simulink model "Custom_SP_inverse"  (R2020b)
settings: Solver=ode45  StartTime=0.0  StopTime=40  RelTol=1e-3
model workspace (MATLAB code in the model file):
  | %% PARAMETERS FOR CUSTOM_SP
  | %%%%%%%%%%%%%%%%%%%%% DENSITY %%%%%%%%%%%%%%%%%%%%%%%
  | al = 2.07; % g/cm^3
  | steel = 7.833; %g/cm^3
  | 
  | %%%%%%%%%%%%%%%%%%%%% BASE COORDINATES %%%%%%%%%%%%%%%%%%%%%%%
  | % Outside coordinates
  | out_base_right = [-335 -170.32; -315 -204.96;
  |     -315 -295.6; -98.49 -420.6; -20 -375.28;
  |     20 -375.28; 315 -204.96; 335 -170.32; 413.49 -125];
  | out_base_left = [413.49 125; 335 170.32;
  |     315 204.96; 20 375.28; -20 375.28;
  |     -98.49 420.6; -315 295.6; -315 204.96; -335 170.32;
  |     -335 -170.32];
  | out_base = [out_base_right; out_base_left];
  | 
  | % Inside coordinates
  | in_base = [-230 -246.52; -230 246.52; -98.49 322.45; 328.49 75.93;
  |     328.49 -75.93; -98.49 -322.45; -230 -246.52];
  | 
  | tot_base = [out_base; in_base];
  | 
  | %%%%%%%%%%%%%%%%%%%%%%% PLATE POSE ON BASE %%%%%%%%%%%%%%%%%%%%%%%%%%%
  | % PLATE POSITION ON BASE
  | plate_1 = [-272.22 -252.09 0];
  | plate_2 = [-82.21 -361.79 0];
  | plate_3 = [354.42 -109.71 0];
  | plate_4 = [354.42 109.71 0];
  | plate_5 = [-82.21 361.79 0];
  | plate_6 = [-272.22  252.09 0];
  | 
  | % ANGLE FOR JOINT ON BASE
  | plate_angle_1 = 0 + pi/2;
  | plate_angle_2 = 2*pi/3 + pi/2;
  | plate_angle_3 = 2*pi/3 + pi/2;
  | plate_angle_4 = 4*pi/3 + pi/2;
  | plate_angle_5 = 4*pi/3 + pi/2;
  | plate_angle_6 = 0 + pi/2;
  | 
  | %%%%%%%%%%%%%%%%%%%%%%%% FLANGE COORDINATES %%%%%%%%%%%%%%%%%%%%%%%%%%%%
  | flange_body = [ -20 22.5; -20 -22.5; 13.6488 -9.3106];
  | 
  | C = linspace(-68.6, 68.6, 21)';
  | C = deg2rad(C);
  | flange_round = [10+10*cos(C) 10*sin(C)];
  | 
  | C = linspace(3*pi/2, -pi/2, 100)';
  | flange_hole = [10+6*cos(C) 6*sin(C)];
  | 
  | flange = [flange_round; flange_body; flange_hole];
  | 
  | %plot(flange(:,1),flange(:,2), 'Color', [0.6 0.6 0.6], 'Marker', '.',...
  | %'MarkerSize', 9, 'MarkerEdgeColor', [1 0 0]);
  | 
  | %%%%%%%%%%%%%%%%%%%%%%%%%%%%% LID %%%%%%%%%%%%%%%%%%%%%%%%%%%%%%
  | % LID COORDINATES
  | C = linspace(-150 , -70, 9)';
  | C = deg2rad(C);
  | lid_round1 = [-171.37+10*cos(C) -103.18+10*sin(C)];
  | 
  | C = linspace(110, 60, 9)';
  | C = deg2rad(C);
  | lid_round2 = [-118.05+10*cos(C) -105.05+10*sin(C)];
  | 
  | C = linspace(60, 10, 9)';
  | C = deg2rad(C);
  | lid_round3 = [-117.46+10*cos(C) -105.39+10*sin(C)];
  | 
  | C = linspace(110, 60, 9)';
  | C = deg2rad(C);
  | lid_round4 = [-32.54+10*cos(C) -154.42+10*sin(C)];
  | 
  | C = linspace(60, 10, 9)';
  | C = deg2rad(C);
  | lid_round5 = [-31.95+10*cos(C) -154.76+10*sin(C)];
  | 
  | C = linspace(-90-80, -90, 9)';
  | C = deg2rad(C);
  | lid_round6 = [-3.67+10*cos(C) -200+10*sin(C)];
  | 
  | C = linspace(-30, 50, 9)';
  | C = deg2rad(C);
  | lid_round7 = [175.04+10*cos(C) -96.82+10*sin(C)];
  | 
  | C = linspace(-140, -90, 9)';
  | C = deg2rad(C);
  | lid_round8 = [150+10*sin(C) -49.71+10*cos(C)];
  | 
  | C = linspace(-90, -40, 9)';
  | C = deg2rad(C);
  | lid_round9 = [150+10*sin(C) -49.03+10*cos(C)];
  | 
  | C = linspace(-140, -90, 9)';
  | C = deg2rad(C);
  | lid_round10 = [150+10*sin(C) 49.03+10*cos(C)];
  | 
  | C = linspace(-90, -40, 9)';
  | C = deg2rad(C);
  | lid_round11 = [150+10*sin(C) 49.71+10*cos(C)];
  | 
  | C = linspace(-50, 30, 9)';
  | C = deg2rad(C);
  | lid_round12 = [175.04+10*cos(C) 96.82+10*sin(C)];
  | 
  | C = linspace(90, 90+80, 9)';
  | C = deg2rad(C);
  | lid_round13 = [-3.67+10*cos(C) 200+10*sin(C)];
  | 
  | C = linspace(-10, -60, 9)';
  | C = deg2rad(C);
  | lid_round14 = [-31.95+10*cos(C) 154.76+10*sin(C)];
  | 
  | C = linspace(-60, -110, 9)';
  | C = deg2rad(C);
  | lid_round15 = [-32.54+10*cos(C) 154.42+10*sin(C)];
  | 
  | C = linspace(-10, -60, 9)';
  | C = deg2rad(C);
  | lid_round16 = [-117.46+10*cos(C) 105.39+10*sin(C)];
  | 
  | C = linspace(-60, -110, 9)';
  | C = deg2rad(C);
  | lid_round17 = [-118.05+10*cos(C) 105.05+10*sin(C)];
  | 
  | C = linspace(70 , 150, 9)';
  | C = deg2rad(C);
  | lid_round18 = [-171.37+10*cos(C) 103.18+10*sin(C)];
  | 
  | lid = [-200 -73.59; lid_round1; lid_round2;
  |     lid_round3;
  |     -100.49 -144.05; -74.51 -159.05; lid_round4;
  |     lid_round5; lid_round6; 36.27 -210; 163.73 -136.41;
  |     lid_round7; lid_round8; lid_round9; 175 -15; 175 15;
  |     lid_round10; lid_round11; lid_round12; 163.73 136.41;
  |     36.27 210; lid_round13; lid_round14; lid_round15;
  |     -74.51 159.05; -100.49 144.05; lid_round16;
  |     lid_round17; lid_round18; -200 73.59];
  | 
  | lid = [-200 -73.59; lid_round1; lid_round2; lid_round3;
  |     -100.49 -144.05; -74.51 -159.05;
  |     lid_round4; lid_round5; lid_round6;
  |     36.27 -210; 163.73 -136.41;
  |     lid_round7; lid_round8; lid_round9;
  |     175 -15; 175 15;
  |     lid_round10; lid_round11; lid_round12;
  |     163.73 136.41; 36.27 210;
  |     lid_round13; lid_round14; lid_round15;
  |     -74.51 159.05; -100.49 144.05;
  |     lid_round16; lid_round17; lid_round18; -200 73.59];
  | 
  | % LID CONNECTOR
  | C = linspace(-150 , -50, 15)';
  | C = deg2rad(C);
  | lid_connector_round1 = [2.15+10*cos(C) -79.37+10*sin(C)];
  | 
  | C = linspace(-50 , 0, 15)';
  | C = deg2rad(C);
  | lid_connector_round2 = [37.5+10*cos(C) -49.71+10*sin(C)];
  | 
  | C = linspace(0 , 50, 15)';
  | C = deg2rad(C);
  | lid_connector_round3 = [37.5+10*cos(C) -49.03+10*sin(C)];
  | 
  | C = linspace(-50, 0, 15)';
  | C = deg2rad(C);
  | lid_connector_round4 = [37.5+10*cos(C) 49.03+10*sin(C)];
  | 
  | C = linspace(0, 50, 15)';
  | C = deg2rad(C);
  | lid_connector_round5 = [37.5+10*cos(C) 49.71+10*sin(C)];
  | 
  | C = linspace(50 , 150, 15)';
  | C = deg2rad(C);
  | lid_connector_round6 = [2.15+10*cos(C) 79.37+10*sin(C)];
  | 
  | lid_connector = [-12.5 -74; lid_connector_round1;
  |     lid_connector_round2; lid_connector_round3; 12.5 -15;
  |     12.5 15; lid_connector_round4; lid_connector_round5;
  |     lid_connector_round6; -12.5 74];
  | 
  | %%%%%%%%%%%%%%%%%%%%%%%%% BALL JOINT %%%%%%%%%%%%%%%%%%%%%%%%%%%
  | % BALL JOINTS
  | C = linspace(138.59, 41.41, 50)';
  | C = deg2rad(C);
  | ball_round = [10*sin(C) 10*cos(C)];
  | 
  | ball_joint = [6 -7.5; ball_round; 6 7.5];
  | 
  | % BALL CONNECTOR
  | C = linspace(-109.47, -70.53, 49)';
  | C = deg2rad(C);
  | ball_round_out = [-16*sin(C) 16*cos(C)];
  | 
  | C = linspace(-57.75, -122.25, 49)';
  | C = deg2rad(C);
  | ball_round_in = [-10*sin(C) 10*cos(C)];
  | 
  | ball_connector = [ball_round_out; ball_round_in];
  | 
  | %%%%%%%%%%%%%%%%%%%%%%%%%% MOTOR %%%%%%%%%%%%%%%%%%%%%%%%%%%
  | % KNOB UNDER MOTOR
  | C = linspace(-90+25.84, -90+64.16, 50)';
  | C = deg2rad(C);
  | knob_under_round1 = [7.5*sin(C) -7.5*cos(C)];
  | 
  | C = linspace( -64.16, -25.84, 50)';
  | C = deg2rad(C);
  | knob_under_round2 = [7.5*cos(C) 7.5*sin(C)];
  | 
  | C = linspace( 25.84, 64.16, 50)';
  | C = deg2rad(C);
  | knob_under_round3 = [7.5*cos(C) 7.5*sin(C)];
  | 
  | C = linspace( 64.16, 25.84, 50)';
  | C = deg2rad(C);
  | knob_under_round4 = [-7.5*cos(C) 7.5*sin(C)];
  | 
  | knob_under = [knob_under_round1; knob_under_round2;
  |     knob_under_round3; knob_under_round4];
  | 
  | % MOTOR UNDER
  | C = linspace(-90, -49, 10)';
  | C = deg2rad(C);
  | knob_under_round1 = [-(19+17)+5.5*sin(C) -11.13-5.5*cos(C)];
  | 
  | C = linspace(-49, 0, 10)';
  | C = deg2rad(C);
  | knob_under_round2 = [-(17+14.77)+5.5*sin(C) -16-5.5*cos(C)];
  | 
  | C = linspace(0, 180, 49)';
  | C = deg2rad(C);
  | knob_under_round3 = [20+21.5*sin(C) -21.5*cos(C)];
  | 
  | C = linspace(180, 180+49, 10)';
  | C = deg2rad(C);
  | knob_under_round4 = [-(17+14.77)+5.5*sin(C) 16-5.5*cos(C)];
  | 
  | C = linspace(270-49, 270, 10)';
  | C = deg2rad(C);
  | knob_under_round5 = [-(19+17)+5.5*sin(C) 11.13-5.5*cos(C)];
  | 
  | motor_under = [knob_under_round1; knob_under_round2;
  |     knob_under_round3; knob_under_round4; knob_under_round5];
  | 
  | % MOTOR LINEAR
  | C = linspace(-180, -101.99, 10)';
  | C = deg2rad(C);
  | motor_top_round1 = [-15.28+3*cos(C) -8.62+3*sin(C)];
  | 
  | C = linspace(-101.99, 101.99, 49)';
  | C = deg2rad(C);
  | motor_top_round2 = [3.12+15.25*cos(C) 15.25*sin(C)];
  | 
  | C = linspace(101.99, 180, 10)';
  | C = deg2rad(C);
  | motor_top_round3 = [-15.28+3*cos(C) 8.62+3*sin(C)];
  | 
  | C = linspace(180, -180, 50)';
  | C = deg2rad(C);
  | motor_top_hole = [3.12+10.1*cos(C) 10.1*sin(C)];
  | 
  | motor_linear = [motor_top_round1; motor_top_round2; motor_top_round3;
  |     -15.28-3 -8.62; motor_top_hole];
  | 
  | %%%%%%%%%%%%%%%%%%%%% MALE %%%%%%%%%%%%%%%%%%%%%%%%%%%
  | male = [15.1 -16; 15.1 16; 10.1 16;
  |     10.1 -11; 6 -11; 6 -16];
  | 
  | %%%%%%%%%%%%%%%%%%%%% FEMALE %%%%%%%%%%%%%%%%%%%%%%%%%
  | female = [15 -19; 15 19; 9.5 19; 9.5 1;
  |     5.055 1; 5.055 -19];
  | 
  | %%%%%%%%%%%%%%%%%%%%% STRAIN GAUGE %%%%%%%%%%%%%%%%%%%%%%
  | strain_gauge = [-38.1 -25.4; -22.4 -25.4; -22.4 11.6;
  |     -13.9 11.6; -13.9 -25.4; 38.1 -25.4; 38.1 25.4;
  |     22.4 25.4; 22.4 -11.6; 13.9 -11.6;
  |     13.9 25.4; -38.1 25.4];
  | 
  | %%%%%%%%%%%%%%%%%%%%% M12 STUFF %%%%%%%%%%%%%%%%%%%%%%%%%%%
  | % M12 BOLT
  | m12_bolt = [0 -18.5; 6 -18.5; 6 11.5; 10.1 11.5; 10.1 18.5; 0 18.5];
  | 
  | % M12 NUT
  | C = linspace(3*pi, pi, 50)';
  | m12_hole = [6*cos(C) 6*sin(C)];
  | m12_nut = [-21.2/2 0; -5.48 -9.5; 5.48 -9.5; 21.2/2 0; 5.48 9.5; -5.48 9.5; -21.2/2 0; m12_hole];
  | 
  | % M12 WASHER
  | m12_washer = [6 -1; 23.5/2 -1; 23.5/2 1; 6 1];
  | 
  | %%%%%%%%%%%%%%%%%%%%%% PLATFORM COORDINATES %%%%%%%%%%%%%%%%%%%%%%%%%%%
  | % Outside coordinates
  | out_platform = [36.27 -210; 163.73 -136.41;
  |     200 -73.59; 200 73.59; 163.73 136.41;
  |     36.27 210; -36.27 210; -163.73 136.41;
  |     -200 73.59; -200 -73.54; -163.73 -136.41; -36.27 -210;
  |     36.27 -210];
  | C = linspace(3*pi/2, -pi/2, 100)';
  | platform_hole = [140*cos(C) 140*sin(C)];
  | platform = [out_platform; platform_hole];
  | 
  | %%%%%%%%%%%%%%%%%%%% STUMP %%%%%%%%%%%%%%%%%%%%%%%
  | C = linspace(-pi/2, -deg2rad(12.47), 100)';
  | stump_round = [70*cos(C) -100+70*sin(C)];
  | stump = [stump_round; 100 170; 0 170];
  | 
  | %% POSITION OF BASE JOINT AND PLATFORM JOINT FOR INVERSE KINEMATICS
  | % BASE JOINT POSITION
  | 
  | zb = 5 + 5 + 30;
  | B = [plate_1(1,1:2) zb; plate_2(1,1:2) zb; plate_3(1,1:2) zb; plate_4(1,1:2) zb; plate_5(1,1:2) zb; plate_6(1,1:2) zb]';
  | 
  | 
  | % JOINT POSITION ON PLATFORM
  | Rot = [cos(deg2rad(120)) -sin(deg2rad(120)); sin(deg2rad(120)) cos(deg2rad(120))];
  | platform_joint_1 = [-200.54-18.5 -48.83]';
  | platform_joint_6 = [-200.54-18.5 48.83]';
  | platform_joint_2 = Rot*platform_joint_6;
  | platform_joint_3 = Rot*platform_joint_1;
  | platform_joint_4 = Rot*platform_joint_2;
  | platform_joint_5 = Rot*platform_joint_3;
  | 
  | % LEG LENGHT AT HOME POSITION
  | %ball_joint_bottom_length = 13.75; %mm
  | %nut_washer = 10 + 2 + 7.25; %mm
  | %female_length = 38 + 2; %mm
  | %motor_length = 58.5 + 163.5; %mm
  | %extender_length = 20 + 50; %mm
  | %male_bolt_nut = 5 + 7 + 25; %mm
  | %strain_gauge_length = 38.1*2; %mm
  | %nut = 10 + 7.25; %mm
  | %ball_joint_top_length = 13.75; %mm
  | 
  | %leg_initial_length = ball_joint_bottom_length + nut_washer + female_length + motor_length + extender_length + male_bolt_nut + strain_gauge_length + nut + ball_joint_top_length;
  | 
  | %height_home = sqrt(leg_initial_length^2 - (plate_1(1)-platform_joint_1(1))^2 - (plate_1(2)-platform_joint_1(2))^2)+zb;
  | height_home = 503.318 + 2.5;
  | leg_initial_length = sqrt((plate_1(1)-platform_joint_1(1))^2 + (plate_1(2)-platform_joint_1(2))^2 + (height_home-zb)^2);
  | P = [platform_joint_1' height_home; platform_joint_2' height_home; platform_joint_3' height_home; platform_joint_4' height_home; platform_joint_5' height_home; platform_joint_6' height_home]';
libraries: nesl_utility x19, Custom_SP_lib x8, sm_lib x2
(part 2 of 2)

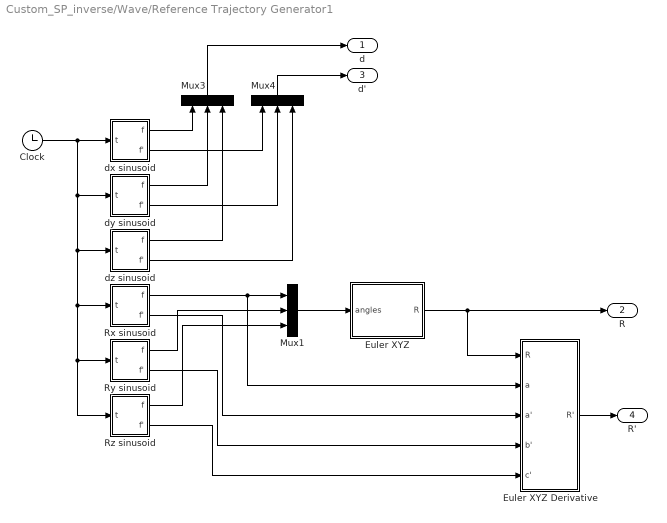
== system Custom_SP_inverse/Wave/Reference Trajectory Generator1 ==
  Clock : Clock
  Euler XYZ : Subsystem  mask(Euler XYZ){}
      mask help: Converts a set of Euler angles to the corresponding rotation matrix from rotated frame to fixed frame coordinates.
      mask Help:
      | An <em>Euler XYZ</em>  block converts a set of Euler angles to the corresponding
      |   rotation matrix from rotated frame to fixed frame coordinates.
      | 
      | Arbitrary 3-D rotations can be parameterized by a vector of three Euler angles:
      |   a, b, and c.  The resulting rotation is given by
      | 
      |     <b>R</b> = <b>R_x</b>(a) <b>R_y</b>(b) <b>R_z</b>(c).
      | 
      | where <b>R_x</b>, <b>R_y</b>, and <b>R_z</b> are rotations about the x, y, and z
      | axes, respectively.
      | 
      | The complete rotation <b>R</b> maps directions from a rotated frame F to a
      | fixed frame G.  Beginning with F and G in an aligned configuration, the full
      | rotation can be realized as a sequence of three rotations: first rotate F
      | about its x-axis, then rotate F about its y-axis, and finally rotate F about its
      | z-axis.  Alternatively, the rotation can be realized in a fixed-frame manner:
      | first rotate F about G's z-axis, then rotate F about G's y-axis, and finally
      | rotate F about G's z-axis.  Both interpretations are correct.
      | 
      | 
      | <h3>Ports</h3>
      | 
      | <ul>
      | 
      | <li> <b>angles</b> The Euler angles a, b, and c (in that order) as a 3-vector
      |   with units of radians.
      | 
      | <li> <b>R</b> The resulting rotation matrix.  This matrix is always a 3 x 3
      | orthogonal matrix with a +1 determinant.
      | 
      | </ul>
  Euler XYZ Derivative : Subsystem  mask(Euler XYZ Derivative){}
      mask help: Computes the first time derivative of a rotation matrix specified by a set of Euler angles.
      mask Help:
      | An <em>Euler XYZ Derivative</em>  block computes the first time derivative of a
      |  rotation matrix specified by a set of Euler angles.
      | 
      | Arbitrary 3-D rotations can be parameterized by a vector of three Euler angles:
      |   a, b, and c.  The resulting rotation is given by
      | 
      |     <b>R</b> = <b>R_x</b>(a) <b>R_y</b>(b) <b>R_z</b>(c).
      | 
      | where <b>R_x</b>, <b>R_y</b>, and <b>R_z</b> are rotations about the x, y, and z
      | axes, respectively.
      | 
      | If a, b, and c are, in turn, functions of time, with instantaneous derivatives
      | a', b', and c', then <b>R'</b>, the time derivative of <b>R</b> is given by
      | 
      |     <b>R'</b> = a' <b>i~ R_x</b>(a) <b>R_y</b>(b) <b>R_z</b>(c) + b' <b>R_x</b>(a) <b>j~ R_y</b>(b) <b>R_z</b>(c) + c' <b>R_x</b>(a) <b>R_y</b>(b) <b>k~ R_z</b>(c),
      | 
      | where <b>~</b> is the canonical operator converting a 3-vector <b>v</b> into a
      | corresponding 3 x 3 skew-symmetric matrix <b>v~</b> such that
      | 
      |     <b>v~ u</b> = <b>v</b> x <b>u</b> for all <b>u</b>.
      | 
      | With some vector algebra, the above expression of <b>R'</b> can be simplified to
      | 
      |     <b>R'</b> = [a' <b>i</b> + b' <b>R_x</b>(a) <b>j</b> ]<b>~</b> <b>R</b> + c' <b>[+R_2, -R_1, 0]</b>
      | 
      | where <b>R_i</b> is the ith column of <b>R</b>.
      | 
      | The block computes the value of <b>R'</b> according to the last equation above.
      | In addition to <b>R</b>, the computation requires the scalar Euler
      | angle <em>a</em>, and the time derivatives of all three Euler angles.
      | 
      | 
      | <h3>Ports</h3>
      | 
      | <ul>
      | 
      | <li> <b>R</b> The rotation matrix defined by the Euler angles <em>a, b,</em>
      | and <em>c</em> (see above).
      | 
      | <li> <b>a</b> The Euler angle corresponding to rotation about the x-axis.
      | 
      | <li> <b>a'</b> The time derivative of the Euler angle corresponding to rotation
      | about the x-axis.
      | 
      | <li> <b>b'</b> The time derivative of the Euler angle corresponding to rotation
      | about the y-axis.
      | 
      | <li> <b>c'</b> The time derivative of the Euler angle corresponding to rotation
      | about the z-axis.
      | 
      | </ul>
  Mux1 : Mux  Inputs=3
  Mux3 : Mux  Inputs=3
  Mux4 : Mux  Inputs=3
  Rx sinusoid : Subsystem  mask(Sinusoidal Trajectory){A=Aa * pi/180, w=wa, p=pa, k=ka * pi/180}
      mask prompts: A "Amplitude"; w "Frequency (deg / s)"; p "Phase (deg)"; k "Offset"
      mask help: Produces a time-varying sinusoid parameterized by amplitude, frequency, phase, and offset. Also produces the first time derivative of this function.
      mask Help:
      | A <em>Sinusoidal Trajectory</em> produces a time-varying sinusoid
      |  parameterized by amplitude, frequency, phase, and offset.  It also produces the
      |  first time derivative of this function.
      | 
      | <h3>Sinsoidal Functions</h3>
      | 
      | An arbitrary sinusoidal function of time and its first time derivative are given by
      | 
      |     f(t) = A sin (w t + p) + k
      |     f'(t) = w A cos (w t + p),
      | 
      | where <em>t</em> is time, and <em>A, w, p,</em> and <em>k</em> are scalar
      | constants.  Given time as an input signal, this block provides the f(t) and
      | f'(t) signals based on the parameters described above.
      | 
      | 
      | <h3>Parameters</h3>
      | 
      | The four parameters specify the scalar parameters described above:
      | 
      | <ul>
      | 
      | <li> <b>A</b> The <em>amplitude</em> of the sinusoid.
      | 
      | <li> <b>w</b> The <em>angular frequency</em> of the sinusoid.
      | 
      | <li> <b>p</b> The <em>phase</em> of the sinusoid.
      | 
      | <li> <b>k</b> The <em>offset</em> of the sinusoid.
      | 
      | </ul>
      | 
      | </ul>
      | 
      | <h3>Ports</h3>
      | 
      | <ul>
      | 
      | <li><b>t</b> The time function, provided as an input signal.
      | 
      | <li><b>f</b> The sinusoid f(t), as described above, as an output signal.
      | 
      | <li><b>f'</b> The sinusoid's first time derivative f'(t), as described above, as an output signal.
      | 
      | </ul>
  Ry sinusoid : Subsystem  mask(Sinusoidal Trajectory){A=Ab * pi/180, w=wb, p=pb, k=kb * pi/180}
      mask prompts: A "Amplitude"; w "Frequency (deg / s)"; p "Phase (deg)"; k "Offset"
      mask help: Produces a time-varying sinusoid parameterized by amplitude, frequency, phase, and offset. Also produces the first time derivative of this function.
      mask Help:
      | A <em>Sinusoidal Trajectory</em> produces a time-varying sinusoid
      |  parameterized by amplitude, frequency, phase, and offset.  It also produces the
      |  first time derivative of this function.
      | 
      | <h3>Sinsoidal Functions</h3>
      | 
      | An arbitrary sinusoidal function of time and its first time derivative are given by
      | 
      |     f(t) = A sin (w t + p) + k
      |     f'(t) = w A cos (w t + p),
      | 
      | where <em>t</em> is time, and <em>A, w, p,</em> and <em>k</em> are scalar
      | constants.  Given time as an input signal, this block provides the f(t) and
      | f'(t) signals based on the parameters described above.
      | 
      | 
      | <h3>Parameters</h3>
      | 
      | The four parameters specify the scalar parameters described above:
      | 
      | <ul>
      | 
      | <li> <b>A</b> The <em>amplitude</em> of the sinusoid.
      | 
      | <li> <b>w</b> The <em>angular frequency</em> of the sinusoid.
      | 
      | <li> <b>p</b> The <em>phase</em> of the sinusoid.
      | 
      | <li> <b>k</b> The <em>offset</em> of the sinusoid.
      | 
      | </ul>
      | 
      | </ul>
      | 
      | <h3>Ports</h3>
      | 
      | <ul>
      | 
      | <li><b>t</b> The time function, provided as an input signal.
      | 
      | <li><b>f</b> The sinusoid f(t), as described above, as an output signal.
      | 
      | <li><b>f'</b> The sinusoid's first time derivative f'(t), as described above, as an output signal.
      | 
      | </ul>
  Rz sinusoid : Subsystem  mask(Sinusoidal Trajectory){A=Ac * pi/180, w=wc, p=pc, k=kc * pi/180}
      mask prompts: A "Amplitude"; w "Frequency (deg / s)"; p "Phase (deg)"; k "Offset"
      mask help: Produces a time-varying sinusoid parameterized by amplitude, frequency, phase, and offset. Also produces the first time derivative of this function.
      mask Help:
      | A <em>Sinusoidal Trajectory</em> produces a time-varying sinusoid
      |  parameterized by amplitude, frequency, phase, and offset.  It also produces the
      |  first time derivative of this function.
      | 
      | <h3>Sinsoidal Functions</h3>
      | 
      | An arbitrary sinusoidal function of time and its first time derivative are given by
      | 
      |     f(t) = A sin (w t + p) + k
      |     f'(t) = w A cos (w t + p),
      | 
      | where <em>t</em> is time, and <em>A, w, p,</em> and <em>k</em> are scalar
      | constants.  Given time as an input signal, this block provides the f(t) and
      | f'(t) signals based on the parameters described above.
      | 
      | 
      | <h3>Parameters</h3>
      | 
      | The four parameters specify the scalar parameters described above:
      | 
      | <ul>
      | 
      | <li> <b>A</b> The <em>amplitude</em> of the sinusoid.
      | 
      | <li> <b>w</b> The <em>angular frequency</em> of the sinusoid.
      | 
      | <li> <b>p</b> The <em>phase</em> of the sinusoid.
      | 
      | <li> <b>k</b> The <em>offset</em> of the sinusoid.
      | 
      | </ul>
      | 
      | </ul>
      | 
      | <h3>Ports</h3>
      | 
      | <ul>
      | 
      | <li><b>t</b> The time function, provided as an input signal.
      | 
      | <li><b>f</b> The sinusoid f(t), as described above, as an output signal.
      | 
      | <li><b>f'</b> The sinusoid's first time derivative f'(t), as described above, as an output signal.
      | 
      | </ul>
  dx sinusoid : Subsystem  mask(Sinusoidal Trajectory){A=Ax, w=wx, p=px, k=kx}
      mask prompts: A "Amplitude"; w "Frequency (deg / s)"; p "Phase (deg)"; k "Offset"
      mask help: Produces a time-varying sinusoid parameterized by amplitude, frequency, phase, and offset. Also produces the first time derivative of this function.
      mask Help:
      | A <em>Sinusoidal Trajectory</em> produces a time-varying sinusoid
      |  parameterized by amplitude, frequency, phase, and offset.  It also produces the
      |  first time derivative of this function.
      | 
      | <h3>Sinsoidal Functions</h3>
      | 
      | An arbitrary sinusoidal function of time and its first time derivative are given by
      | 
      |     f(t) = A sin (w t + p) + k
      |     f'(t) = w A cos (w t + p),
      | 
      | where <em>t</em> is time, and <em>A, w, p,</em> and <em>k</em> are scalar
      | constants.  Given time as an input signal, this block provides the f(t) and
      | f'(t) signals based on the parameters described above.
      | 
      | 
      | <h3>Parameters</h3>
      | 
      | The four parameters specify the scalar parameters described above:
      | 
      | <ul>
      | 
      | <li> <b>A</b> The <em>amplitude</em> of the sinusoid.
      | 
      | <li> <b>w</b> The <em>angular frequency</em> of the sinusoid.
      | 
      | <li> <b>p</b> The <em>phase</em> of the sinusoid.
      | 
      | <li> <b>k</b> The <em>offset</em> of the sinusoid.
      | 
      | </ul>
      | 
      | </ul>
      | 
      | <h3>Ports</h3>
      | 
      | <ul>
      | 
      | <li><b>t</b> The time function, provided as an input signal.
      | 
      | <li><b>f</b> The sinusoid f(t), as described above, as an output signal.
      | 
      | <li><b>f'</b> The sinusoid's first time derivative f'(t), as described above, as an output signal.
      | 
      | </ul>
  dy sinusoid : Subsystem  mask(Sinusoidal Trajectory){A=Ay, w=wy, p=py, k=ky}
      mask prompts: A "Amplitude"; w "Frequency (deg / s)"; p "Phase (deg)"; k "Offset"
      mask help: Produces a time-varying sinusoid parameterized by amplitude, frequency, phase, and offset. Also produces the first time derivative of this function.
      mask Help:
      | A <em>Sinusoidal Trajectory</em> produces a time-varying sinusoid
      |  parameterized by amplitude, frequency, phase, and offset.  It also produces the
      |  first time derivative of this function.
      | 
      | <h3>Sinsoidal Functions</h3>
      | 
      | An arbitrary sinusoidal function of time and its first time derivative are given by
      | 
      |     f(t) = A sin (w t + p) + k
      |     f'(t) = w A cos (w t + p),
      | 
      | where <em>t</em> is time, and <em>A, w, p,</em> and <em>k</em> are scalar
      | constants.  Given time as an input signal, this block provides the f(t) and
      | f'(t) signals based on the parameters described above.
      | 
      | 
      | <h3>Parameters</h3>
      | 
      | The four parameters specify the scalar parameters described above:
      | 
      | <ul>
      | 
      | <li> <b>A</b> The <em>amplitude</em> of the sinusoid.
      | 
      | <li> <b>w</b> The <em>angular frequency</em> of the sinusoid.
      | 
      | <li> <b>p</b> The <em>phase</em> of the sinusoid.
      | 
      | <li> <b>k</b> The <em>offset</em> of the sinusoid.
      | 
      | </ul>
      | 
      | </ul>
      | 
      | <h3>Ports</h3>
      | 
      | <ul>
      | 
      | <li><b>t</b> The time function, provided as an input signal.
      | 
      | <li><b>f</b> The sinusoid f(t), as described above, as an output signal.
      | 
      | <li><b>f'</b> The sinusoid's first time derivative f'(t), as described above, as an output signal.
      | 
      | </ul>
  dz sinusoid : Subsystem  mask(Sinusoidal Trajectory){A=Az, w=wz, p=pz, k=kz}
      mask prompts: A "Amplitude"; w "Frequency (deg / s)"; p "Phase (deg)"; k "Offset"
      mask help: Produces a time-varying sinusoid parameterized by amplitude, frequency, phase, and offset. Also produces the first time derivative of this function.
      mask Help:
      | A <em>Sinusoidal Trajectory</em> produces a time-varying sinusoid
      |  parameterized by amplitude, frequency, phase, and offset.  It also produces the
      |  first time derivative of this function.
      | 
      | <h3>Sinsoidal Functions</h3>
      | 
      | An arbitrary sinusoidal function of time and its first time derivative are given by
      | 
      |     f(t) = A sin (w t + p) + k
      |     f'(t) = w A cos (w t + p),
      | 
      | where <em>t</em> is time, and <em>A, w, p,</em> and <em>k</em> are scalar
      | constants.  Given time as an input signal, this block provides the f(t) and
      | f'(t) signals based on the parameters described above.
      | 
      | 
      | <h3>Parameters</h3>
      | 
      | The four parameters specify the scalar parameters described above:
      | 
      | <ul>
      | 
      | <li> <b>A</b> The <em>amplitude</em> of the sinusoid.
      | 
      | <li> <b>w</b> The <em>angular frequency</em> of the sinusoid.
      | 
      | <li> <b>p</b> The <em>phase</em> of the sinusoid.
      | 
      | <li> <b>k</b> The <em>offset</em> of the sinusoid.
      | 
      | </ul>
      | 
      | </ul>
      | 
      | <h3>Ports</h3>
      | 
      | <ul>
      | 
      | <li><b>t</b> The time function, provided as an input signal.
      | 
      | <li><b>f</b> The sinusoid f(t), as described above, as an output signal.
      | 
      | <li><b>f'</b> The sinusoid's first time derivative f'(t), as described above, as an output signal.
      | 
      | </ul>
  d : Outport  VectorParamsAs1DForOutWhenUnconnected=off
  R : Outport  Port=2  VectorParamsAs1DForOutWhenUnconnected=off
  d' : Outport  Port=3  VectorParamsAs1DForOutWhenUnconnected=off
  R' : Outport  Port=4  VectorParamsAs1DForOutWhenUnconnected=off
  wires:
  dx sinusoid/1(f) -> Mux3/1
  dy sinusoid/1(f) -> Mux3/2
  dz sinusoid/1(f) -> Mux3/3
  dx sinusoid/2(f') -> Mux4/1
  dy sinusoid/2(f') -> Mux4/2
  dz sinusoid/2(f') -> Mux4/3
  Mux3/1 -> d/1
  Mux4/1 -> d'/1
  Rx sinusoid/1(f) -> Mux1/1, Euler XYZ Derivative/2(a)
  Euler XYZ Derivative/1(R') -> R'/1
  Clock/1 -> Ry sinusoid/1(t), Rz sinusoid/1(t), Rx sinusoid/1(t), dz sinusoid/1(t), dy sinusoid/1(t), dx sinusoid/1(t)
  Ry sinusoid/1(f) -> Mux1/2
  Rz sinusoid/1(f) -> Mux1/3
  Rx sinusoid/2(f') -> Euler XYZ Derivative/3(a')
  Ry sinusoid/2(f') -> Euler XYZ Derivative/4(b')
  Rz sinusoid/2(f') -> Euler XYZ Derivative/5(c')
  Mux1/1 -> Euler XYZ/1(angles)
  Euler XYZ/1(R) -> R/1, Euler XYZ Derivative/1(R)

== system Custom_SP_inverse/Wave/Inverse Kinematics Module/Norm 1 ==
  v : Inport
  Dot Product : DotProduct  OutDataTypeStr=Inherit: Inherit via internal rule
  Sqrt : Sqrt  SaturateOnIntegerOverflow=on
  ||v|| : Outport  VectorParamsAs1DForOutWhenUnconnected=off
  wires:
  Dot Product/1 -> Sqrt/1
  Sqrt/1 -> ||v||/1
  v/1 -> Dot Product/1, Dot Product/2

== system Custom_SP_inverse/Wave/Inverse Kinematics Module/Norm 2 ==
  v : Inport
  Dot Product : DotProduct  OutDataTypeStr=Inherit: Inherit via internal rule
  Sqrt : Sqrt  SaturateOnIntegerOverflow=on
  ||v|| : Outport  VectorParamsAs1DForOutWhenUnconnected=off
  wires:
  Dot Product/1 -> Sqrt/1
  Sqrt/1 -> ||v||/1
  v/1 -> Dot Product/1, Dot Product/2

== system Custom_SP_inverse/Wave/Inverse Kinematics Module/Norm 3 ==
  v : Inport
  Dot Product : DotProduct  OutDataTypeStr=Inherit: Inherit via internal rule
  Sqrt : Sqrt  SaturateOnIntegerOverflow=on
  ||v|| : Outport  VectorParamsAs1DForOutWhenUnconnected=off
  wires:
  Dot Product/1 -> Sqrt/1
  Sqrt/1 -> ||v||/1
  v/1 -> Dot Product/1, Dot Product/2

== system Custom_SP_inverse/Wave/Inverse Kinematics Module/Norm 4 ==
  v : Inport
  Dot Product : DotProduct  OutDataTypeStr=Inherit: Inherit via internal rule
  Sqrt : Sqrt  SaturateOnIntegerOverflow=on
  ||v|| : Outport  VectorParamsAs1DForOutWhenUnconnected=off
  wires:
  Dot Product/1 -> Sqrt/1
  Sqrt/1 -> ||v||/1
  v/1 -> Dot Product/1, Dot Product/2

== system Custom_SP_inverse/Wave/Inverse Kinematics Module/Norm 5 ==
  v : Inport
  Dot Product : DotProduct  OutDataTypeStr=Inherit: Inherit via internal rule
  Sqrt : Sqrt  SaturateOnIntegerOverflow=on
  ||v|| : Outport  VectorParamsAs1DForOutWhenUnconnected=off
  wires:
  Dot Product/1 -> Sqrt/1
  Sqrt/1 -> ||v||/1
  v/1 -> Dot Product/1, Dot Product/2

== system Custom_SP_inverse/Wave/Inverse Kinematics Module/Norm 6 ==
  v : Inport
  Dot Product : DotProduct  OutDataTypeStr=Inherit: Inherit via internal rule
  Sqrt : Sqrt  SaturateOnIntegerOverflow=on
  ||v|| : Outport  VectorParamsAs1DForOutWhenUnconnected=off
  wires:
  Dot Product/1 -> Sqrt/1
  Sqrt/1 -> ||v||/1
  v/1 -> Dot Product/1, Dot Product/2

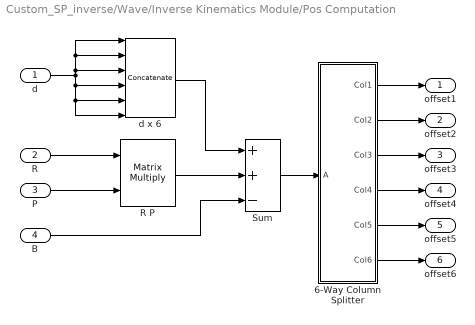
== system Custom_SP_inverse/Wave/Inverse Kinematics Module/Pos Computation ==
  d : Inport
  R : Inport  Port=2
  P : Inport  Port=3
  B : Inport  Port=4
  6-Way Column Splitter : Subsystem
  R P : Product  Multiplication=Matrix(*)  RndMeth=Zero
  Sum : Sum  Inputs=++-
  d x 6 : Concatenate  NumInputs=6  Mode=Multidimensional array  ConcatenateDimension=2
  offset1 : Outport  VectorParamsAs1DForOutWhenUnconnected=off
  offset2 : Outport  Port=2  VectorParamsAs1DForOutWhenUnconnected=off
  offset3 : Outport  Port=3  VectorParamsAs1DForOutWhenUnconnected=off
  offset4 : Outport  Port=4  VectorParamsAs1DForOutWhenUnconnected=off
  offset5 : Outport  Port=5  VectorParamsAs1DForOutWhenUnconnected=off
  offset6 : Outport  Port=6  VectorParamsAs1DForOutWhenUnconnected=off
  wires:
  d/1 -> d x 6/3, d x 6/2, d x 6/1, d x 6/4, d x 6/5, d x 6/6
  Sum/1 -> 6-Way Column Splitter/1(A)
  P/1 -> R P/2
  6-Way Column Splitter/1(Col1) -> offset1/1
  R/1 -> R P/1
  6-Way Column Splitter/2(Col2) -> offset2/1
  6-Way Column Splitter/3(Col3) -> offset3/1
  6-Way Column Splitter/4(Col4) -> offset4/1
  6-Way Column Splitter/5(Col5) -> offset5/1
  6-Way Column Splitter/6(Col6) -> offset6/1
  d x 6/1 -> Sum/1
  B/1 -> Sum/3
  R P/1 -> Sum/2

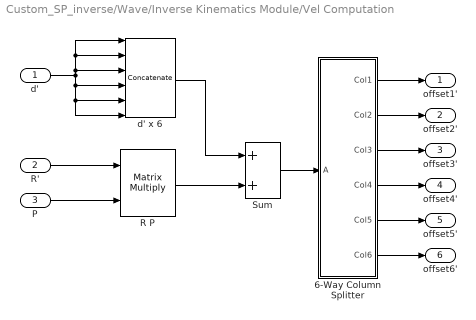
== system Custom_SP_inverse/Wave/Inverse Kinematics Module/Vel Computation ==
  d' : Inport
  R' : Inport  Port=2
  P : Inport  Port=3
  6-Way Column Splitter : Subsystem
  R P : Product  Multiplication=Matrix(*)  RndMeth=Zero
  Sum : Sum
  d' x 6 : Concatenate  NumInputs=6  Mode=Multidimensional array  ConcatenateDimension=2
  offset1' : Outport  VectorParamsAs1DForOutWhenUnconnected=off
  offset2' : Outport  Port=2  VectorParamsAs1DForOutWhenUnconnected=off
  offset3' : Outport  Port=3  VectorParamsAs1DForOutWhenUnconnected=off
  offset4' : Outport  Port=4  VectorParamsAs1DForOutWhenUnconnected=off
  offset5' : Outport  Port=5  VectorParamsAs1DForOutWhenUnconnected=off
  offset6' : Outport  Port=6  VectorParamsAs1DForOutWhenUnconnected=off
  wires:
  d'/1 -> d' x 6/3, d' x 6/2, d' x 6/1, d' x 6/4, d' x 6/5, d' x 6/6
  Sum/1 -> 6-Way Column Splitter/1(A)
  P/1 -> R P/2
  6-Way Column Splitter/1(Col1) -> offset1'/1
  R'/1 -> R P/1
  6-Way Column Splitter/2(Col2) -> offset2'/1
  6-Way Column Splitter/3(Col3) -> offset3'/1
  6-Way Column Splitter/4(Col4) -> offset4'/1
  6-Way Column Splitter/5(Col5) -> offset5'/1
  6-Way Column Splitter/6(Col6) -> offset6'/1
  d' x 6/1 -> Sum/1
  R P/1 -> Sum/2

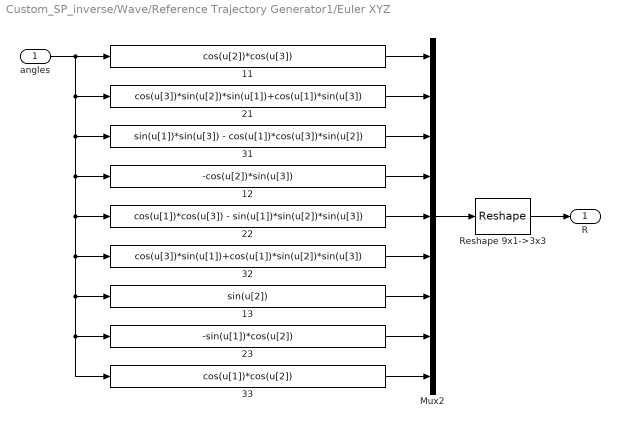
== system Custom_SP_inverse/Wave/Reference Trajectory Generator1/Euler XYZ ==
  angles : Inport
  11 : Fcn  Expr=cos(u[2])*cos(u[3])
  12 : Fcn  Expr=-cos(u[2])*sin(u[3])
  13 : Fcn  Expr=sin(u[2])
  21 : Fcn  Expr=cos(u[3])*sin(u[2])*sin(u[1])+cos(u[1])*sin(u[3])
  22 : Fcn  Expr=cos(u[1])*cos(u[3]) - sin(u[1])*sin(u[2])*sin(u[3])
  23 : Fcn  Expr=-sin(u[1])*cos(u[2])
  31 : Fcn  Expr=sin(u[1])*sin(u[3]) - cos(u[1])*cos(u[3])*sin(u[2])
  32 : Fcn  Expr=cos(u[3])*sin(u[1])+cos(u[1])*sin(u[2])*sin(u[3])
  33 : Fcn  Expr=cos(u[1])*cos(u[2])
  Mux2 : Mux  Inputs=9
  Reshape 9x1->3x3 : Reshape  OutputDimensionality=Customize  OutputDimensions=[3,3]
  R : Outport  VectorParamsAs1DForOutWhenUnconnected=off
  wires:
  angles/1 -> 23/1, 33/1, 13/1, 32/1, 22/1, 12/1, 31/1, 21/1, 11/1
  33/1 -> Mux2/9
  23/1 -> Mux2/8
  13/1 -> Mux2/7
  32/1 -> Mux2/6
  22/1 -> Mux2/5
  12/1 -> Mux2/4
  31/1 -> Mux2/3
  21/1 -> Mux2/2
  11/1 -> Mux2/1
  Mux2/1 -> Reshape 9x1->3x3/1
  Reshape 9x1->3x3/1 -> R/1

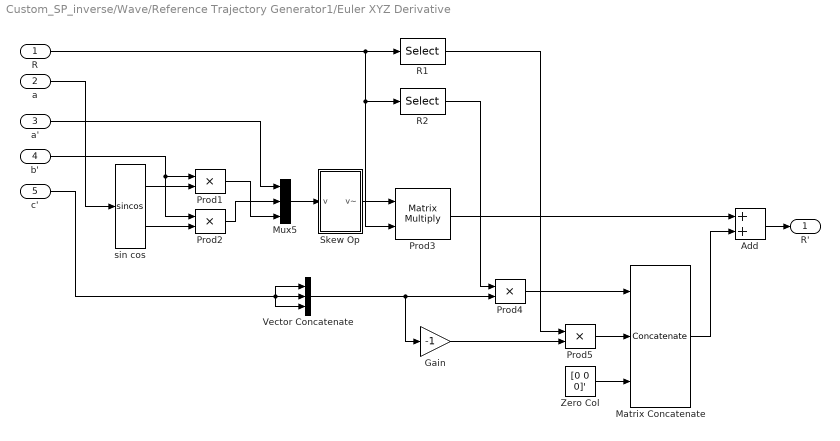
== system Custom_SP_inverse/Wave/Reference Trajectory Generator1/Euler XYZ Derivative ==
  R : Inport
  a : Inport  Port=2
  a' : Inport  Port=3
  b' : Inport  Port=4
  c' : Inport  Port=5
  Add : Sum
  Gain : Gain  Gain=-1
  Matrix Concatenate : Concatenate  NumInputs=3  Mode=Multidimensional array  ConcatenateDimension=2
  Mux5 : Mux  Inputs=3
  Prod{1..2,4..5} (4 alike) : Product  RndMeth=Zero
  Prod3 : Product  Multiplication=Matrix(*)  RndMeth=Zero
  R1 : Selector  NumberOfDimensions=2  InputPortWidth=3  IndexOptions=Select all,Index vector (dialog)  Indices=[1 3],1  OutputSizes=1,1
  R2 : Selector  NumberOfDimensions=2  InputPortWidth=3  IndexOptions=Select all,Index vector (dialog)  Indices=[1 3],2  OutputSizes=1,1
  Skew Op : Subsystem
  Vector Concatenate : Concatenate  NumInputs=3  Mode=Multidimensional array
  Zero Col : Constant  Value=[0 0 0]'
  sin cos : Trigonometry  Operator=sincos
  R' : Outport  VectorParamsAs1DForOutWhenUnconnected=off
  wires:
  a/1 -> sin cos/1
  sin cos/1 -> Prod1/2
  sin cos/2 -> Prod2/2
  b'/1 -> Prod2/1, Prod1/1
  a'/1 -> Mux5/1
  Prod2/1 -> Mux5/2
  Prod1/1 -> Mux5/3
  Mux5/1 -> Skew Op/1(v)
  Vector Concatenate/1 -> Prod4/2, Gain/1
  R2/1 -> Prod4/1
  Gain/1 -> Prod5/2
  Zero Col/1 -> Matrix Concatenate/3
  Prod5/1 -> Matrix Concatenate/2
  Prod4/1 -> Matrix Concatenate/1
  R1/1 -> Prod5/1
  Prod3/1 -> Add/1
  Matrix Concatenate/1 -> Add/2
  Add/1 -> R'/1
  R/1 -> R1/1, Prod3/2, R2/1
  Skew Op/1(v~) -> Prod3/1
  c'/1 -> Vector Concatenate/2, Vector Concatenate/1, Vector Concatenate/3

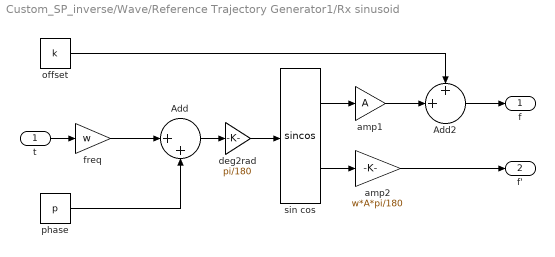
== system Custom_SP_inverse/Wave/Reference Trajectory Generator1/Rx sinusoid ==
  t : Inport
  Add : Sum  Inputs=|++
  Add2 : Sum  Inputs=++|
  amp1 : Gain  Gain=A
  amp2 : Gain  Gain=w*A*pi/180
  deg2rad : Gain  Gain=pi/180
  freq : Gain  Gain=w
  offset : Constant  Value=k  VectorParams1D=off
  phase : Constant  Value=p  VectorParams1D=off
  sin cos : Trigonometry  Operator=sincos
  f : Outport  VectorParamsAs1DForOutWhenUnconnected=off
  f' : Outport  Port=2  VectorParamsAs1DForOutWhenUnconnected=off
  wires:
  t/1 -> freq/1
  Add/1 -> deg2rad/1
  phase/1 -> Add/2
  amp2/1 -> f'/1
  Add2/1 -> f/1
  offset/1 -> Add2/1
  sin cos/1 -> amp1/1
  sin cos/2 -> amp2/1
  amp1/1 -> Add2/2
  freq/1 -> Add/1
  deg2rad/1 -> sin cos/1

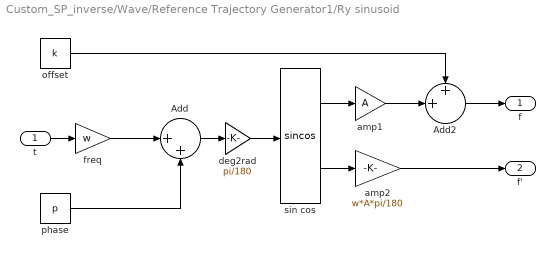
== system Custom_SP_inverse/Wave/Reference Trajectory Generator1/Ry sinusoid ==
  t : Inport
  Add : Sum  Inputs=|++
  Add2 : Sum  Inputs=++|
  amp1 : Gain  Gain=A
  amp2 : Gain  Gain=w*A*pi/180
  deg2rad : Gain  Gain=pi/180
  freq : Gain  Gain=w
  offset : Constant  Value=k  VectorParams1D=off
  phase : Constant  Value=p  VectorParams1D=off
  sin cos : Trigonometry  Operator=sincos
  f : Outport  VectorParamsAs1DForOutWhenUnconnected=off
  f' : Outport  Port=2  VectorParamsAs1DForOutWhenUnconnected=off
  wires:
  t/1 -> freq/1
  Add/1 -> deg2rad/1
  phase/1 -> Add/2
  amp2/1 -> f'/1
  Add2/1 -> f/1
  offset/1 -> Add2/1
  sin cos/1 -> amp1/1
  sin cos/2 -> amp2/1
  amp1/1 -> Add2/2
  freq/1 -> Add/1
  deg2rad/1 -> sin cos/1

== system Custom_SP_inverse/Wave/Reference Trajectory Generator1/Rz sinusoid ==
  t : Inport
  Add : Sum  Inputs=|++
  Add2 : Sum  Inputs=++|
  amp1 : Gain  Gain=A
  amp2 : Gain  Gain=w*A*pi/180
  deg2rad : Gain  Gain=pi/180
  freq : Gain  Gain=w
  offset : Constant  Value=k  VectorParams1D=off
  phase : Constant  Value=p  VectorParams1D=off
  sin cos : Trigonometry  Operator=sincos
  f : Outport  VectorParamsAs1DForOutWhenUnconnected=off
  f' : Outport  Port=2  VectorParamsAs1DForOutWhenUnconnected=off
  wires:
  t/1 -> freq/1
  Add/1 -> deg2rad/1
  phase/1 -> Add/2
  amp2/1 -> f'/1
  Add2/1 -> f/1
  offset/1 -> Add2/1
  sin cos/1 -> amp1/1
  sin cos/2 -> amp2/1
  amp1/1 -> Add2/2
  freq/1 -> Add/1
  deg2rad/1 -> sin cos/1

== system Custom_SP_inverse/Wave/Reference Trajectory Generator1/dx sinusoid ==
  t : Inport
  Add : Sum  Inputs=|++
  Add2 : Sum  Inputs=++|
  amp1 : Gain  Gain=A
  amp2 : Gain  Gain=w*A*pi/180
  deg2rad : Gain  Gain=pi/180
  freq : Gain  Gain=w
  offset : Constant  Value=k  VectorParams1D=off
  phase : Constant  Value=p  VectorParams1D=off
  sin cos : Trigonometry  Operator=sincos
  f : Outport  VectorParamsAs1DForOutWhenUnconnected=off
  f' : Outport  Port=2  VectorParamsAs1DForOutWhenUnconnected=off
  wires:
  t/1 -> freq/1
  Add/1 -> deg2rad/1
  phase/1 -> Add/2
  amp2/1 -> f'/1
  Add2/1 -> f/1
  offset/1 -> Add2/1
  sin cos/1 -> amp1/1
  sin cos/2 -> amp2/1
  amp1/1 -> Add2/2
  freq/1 -> Add/1
  deg2rad/1 -> sin cos/1

== system Custom_SP_inverse/Wave/Reference Trajectory Generator1/dy sinusoid ==
  t : Inport
  Add : Sum  Inputs=|++
  Add2 : Sum  Inputs=++|
  amp1 : Gain  Gain=A
  amp2 : Gain  Gain=w*A*pi/180
  deg2rad : Gain  Gain=pi/180
  freq : Gain  Gain=w
  offset : Constant  Value=k  VectorParams1D=off
  phase : Constant  Value=p  VectorParams1D=off
  sin cos : Trigonometry  Operator=sincos
  f : Outport  VectorParamsAs1DForOutWhenUnconnected=off
  f' : Outport  Port=2  VectorParamsAs1DForOutWhenUnconnected=off
  wires:
  t/1 -> freq/1
  Add/1 -> deg2rad/1
  phase/1 -> Add/2
  amp2/1 -> f'/1
  Add2/1 -> f/1
  offset/1 -> Add2/1
  sin cos/1 -> amp1/1
  sin cos/2 -> amp2/1
  amp1/1 -> Add2/2
  freq/1 -> Add/1
  deg2rad/1 -> sin cos/1

== system Custom_SP_inverse/Wave/Reference Trajectory Generator1/dz sinusoid ==
  t : Inport
  Add : Sum  Inputs=|++
  Add2 : Sum  Inputs=++|
  amp1 : Gain  Gain=A
  amp2 : Gain  Gain=w*A*pi/180
  deg2rad : Gain  Gain=pi/180
  freq : Gain  Gain=w
  offset : Constant  Value=k  VectorParams1D=off
  phase : Constant  Value=p  VectorParams1D=off
  sin cos : Trigonometry  Operator=sincos
  f : Outport  VectorParamsAs1DForOutWhenUnconnected=off
  f' : Outport  Port=2  VectorParamsAs1DForOutWhenUnconnected=off
  wires:
  t/1 -> freq/1
  Add/1 -> deg2rad/1
  phase/1 -> Add/2
  amp2/1 -> f'/1
  Add2/1 -> f/1
  offset/1 -> Add2/1
  sin cos/1 -> amp1/1
  sin cos/2 -> amp2/1
  amp1/1 -> Add2/2
  freq/1 -> Add/1
  deg2rad/1 -> sin cos/1

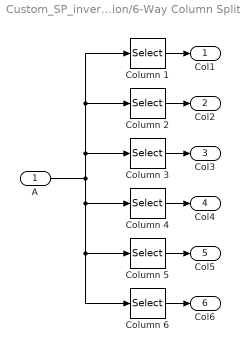
== system Custom_SP_inverse/Wave/Inverse Kinematics Module/Pos Computation/6-Way Column Splitter ==
  A : Inport
  Column 1 : Selector  NumberOfDimensions=2  InputPortWidth=3  IndexOptions=Select all,Index vector (dialog)  Indices=-1,1  OutputSizes=1
  Column 2 : Selector  NumberOfDimensions=2  InputPortWidth=3  IndexOptions=Select all,Index vector (dialog)  Indices=-1,2  OutputSizes=1
  Column 3 : Selector  NumberOfDimensions=2  InputPortWidth=3  IndexOptions=Select all,Index vector (dialog)  Indices=-1,3  OutputSizes=1
  Column 4 : Selector  NumberOfDimensions=2  InputPortWidth=3  IndexOptions=Select all,Index vector (dialog)  Indices=-1,4  OutputSizes=1
  Column 5 : Selector  NumberOfDimensions=2  InputPortWidth=3  IndexOptions=Select all,Index vector (dialog)  Indices=-1,5  OutputSizes=1
  Column 6 : Selector  NumberOfDimensions=2  InputPortWidth=3  IndexOptions=Select all,Index vector (dialog)  Indices=-1,6  OutputSizes=1
  Col1 : Outport  VectorParamsAs1DForOutWhenUnconnected=off
  Col2 : Outport  Port=2  VectorParamsAs1DForOutWhenUnconnected=off
  Col3 : Outport  Port=3  VectorParamsAs1DForOutWhenUnconnected=off
  Col4 : Outport  Port=4  VectorParamsAs1DForOutWhenUnconnected=off
  Col5 : Outport  Port=5  VectorParamsAs1DForOutWhenUnconnected=off
  Col6 : Outport  Port=6  VectorParamsAs1DForOutWhenUnconnected=off
  wires:
  A/1 -> Column 3/1, Column 2/1, Column 1/1, Column 4/1, Column 5/1, Column 6/1
  Column 1/1 -> Col1/1
  Column 2/1 -> Col2/1
  Column 3/1 -> Col3/1
  Column 4/1 -> Col4/1
  Column 5/1 -> Col5/1
  Column 6/1 -> Col6/1

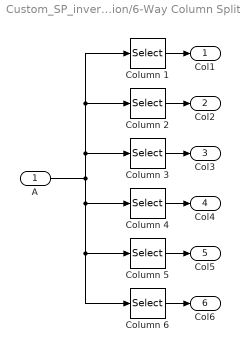
== system Custom_SP_inverse/Wave/Inverse Kinematics Module/Vel Computation/6-Way Column Splitter ==
  A : Inport
  Column 1 : Selector  NumberOfDimensions=2  InputPortWidth=3  IndexOptions=Select all,Index vector (dialog)  Indices=-1,1  OutputSizes=1
  Column 2 : Selector  NumberOfDimensions=2  InputPortWidth=3  IndexOptions=Select all,Index vector (dialog)  Indices=-1,2  OutputSizes=1
  Column 3 : Selector  NumberOfDimensions=2  InputPortWidth=3  IndexOptions=Select all,Index vector (dialog)  Indices=-1,3  OutputSizes=1
  Column 4 : Selector  NumberOfDimensions=2  InputPortWidth=3  IndexOptions=Select all,Index vector (dialog)  Indices=-1,4  OutputSizes=1
  Column 5 : Selector  NumberOfDimensions=2  InputPortWidth=3  IndexOptions=Select all,Index vector (dialog)  Indices=-1,5  OutputSizes=1
  Column 6 : Selector  NumberOfDimensions=2  InputPortWidth=3  IndexOptions=Select all,Index vector (dialog)  Indices=-1,6  OutputSizes=1
  Col1 : Outport  VectorParamsAs1DForOutWhenUnconnected=off
  Col2 : Outport  Port=2  VectorParamsAs1DForOutWhenUnconnected=off
  Col3 : Outport  Port=3  VectorParamsAs1DForOutWhenUnconnected=off
  Col4 : Outport  Port=4  VectorParamsAs1DForOutWhenUnconnected=off
  Col5 : Outport  Port=5  VectorParamsAs1DForOutWhenUnconnected=off
  Col6 : Outport  Port=6  VectorParamsAs1DForOutWhenUnconnected=off
  wires:
  A/1 -> Column 3/1, Column 2/1, Column 1/1, Column 4/1, Column 5/1, Column 6/1
  Column 1/1 -> Col1/1
  Column 2/1 -> Col2/1
  Column 3/1 -> Col3/1
  Column 4/1 -> Col4/1
  Column 5/1 -> Col5/1
  Column 6/1 -> Col6/1

== system Custom_SP_inverse/Wave/Reference Trajectory Generator1/Euler XYZ Derivative/Skew Op ==
  v : Inport
  Demux : Demux  Outputs=3
  Demux1 : Demux  Outputs=3
  Gain : Gain  Gain=-1
  Mux6 : Mux  Inputs=9
  Reshape 9x1->3x3 : Reshape  OutputDimensionality=Customize  OutputDimensions=[3,3]
  Zero : Constant  Value=0
  v~ : Outport  VectorParamsAs1DForOutWhenUnconnected=off
  wires:
  Mux6/1 -> Reshape 9x1->3x3/1
  v/1 -> Demux/1, Gain/1
  Gain/1 -> Demux1/1
  Reshape 9x1->3x3/1 -> v~/1
  Zero/1 -> Mux6/1, Mux6/5, Mux6/9
  Demux/3 -> Mux6/2
  Demux1/2 -> Mux6/3
  Demux1/3 -> Mux6/4
  Demux/1 -> Mux6/6
  Demux/2 -> Mux6/7
  Demux1/1 -> Mux6/8
